simulink model "Motor_EncRead_AnalogRead"  (R2023a)
settings: Solver=ode3  StartTime=0.0  StopTime=inf  RelTol=1e-3  EnableMultiTasking=on
undefined symbols (not defined in the file or in its folder): ticksPerRot, wheelR
libraries: M5Core_Library x4, arduinolib x1
settings Model: ExtModeTrigDuration=2  Creator=auw_a  LastModifiedBy=auw_a
settings SolverCC: AlgebraicLoopSolver=TrustRegion
settings DataIOCC: LimitDataPoints=on  SaveFormat=Array
settings OptimizationCC: ExpressionDepthLimit=2147483647  LifeSpan=Inf  MaxStackSize=64
settings DebuggingCC: UnderspecifiedInitializationDetection=Classic  MergeDetectMultiDrivingBlocksExec=none  FcnCallInpInsideContextMsg=warning  UnconnectedInputMsg=warning  UnconnectedOutputMsg=warning  UnconnectedLineMsg=warning  AllowSymbolicDim=off  StateNameClashWarn=warning  SFUnexpectedBacktrackingDiag=warning  SFNoUnconditionalDefaultTransitionDiag=warning  SFExecutionAtInitializationDiag=none  ArithmeticOperatorsInVariantConditions=warning
settings HardwareCC: ProdBitPerPointer=32  ProdBitPerSizeT=32  ProdBitPerPtrDiffT=32  ProdLargestAtomicInteger=Long  ProdLargestAtomicFloat=Double  ProdWordSize=32  ProdHWDeviceType=ARM Compatible->ARM Cortex
settings ModelReferenceCC: EnableRefExpFcnMdlSchedulingChecks=on  PropagateSignalLabelsOutOfModel=off
settings SFSimCC: SimUseLocalCustomCode=off  CustomCodeUndefinedFunction=UseInterfaceOnly
settings RTWCC: Description=Embedded Coder  SystemTargetFile=ert.tlc  HardwareBoard=ESP32-WROOM(Arduino Compatible)  TemplateMakefile=ert_default_tmf  GenerateReport=on  RTWVerbose=off  RTWUseLocalCustomCode=off  Toolchain=ESP32  BuildConfiguration=Faster Runs  LaunchReport=on
settings CodeAppCC: ForceParamTrailComments=on  OperatorAnnotations=on  StateflowObjectComments=on  MATLABSourceComments=on
settings ERTTargetCC: MultiwordLength=2048  ERTCustomFileBanners=off  SupportContinuousTime=on  SupportNonInlinedSFcns=on  RemoveResetFunc=off  SupportVariableSizeSignals=on  ModelStepFunctionPrototypeControlCompliant=off  ExtModeTransport=3  ExtModeStaticAlloc=on  ExtModeAutomaticAllocSize=off  ExtModeStaticAllocSize=65536  ExtModeMexFile=ext_xcp  ExtModeIntrfLevel=Level2 - Open
settings ConfigComp: CovMetricSettings=dw  CovSaveCumulativeToWorkspaceVar=on  CovSaveSingleToWorkspaceVar=on  CovExternalEMLEnable=off  CovSFcnEnable=off

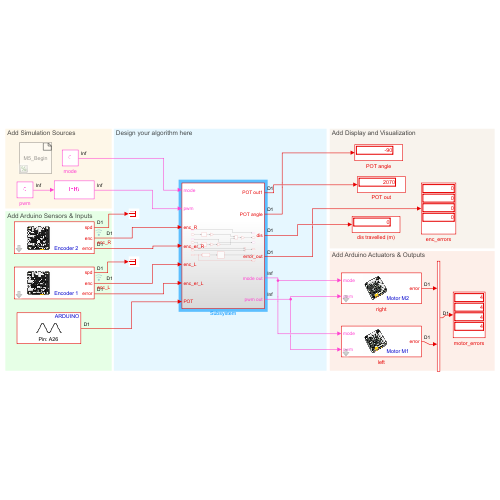
[thumbnail: Simulink's stored preview of the top-level diagram]
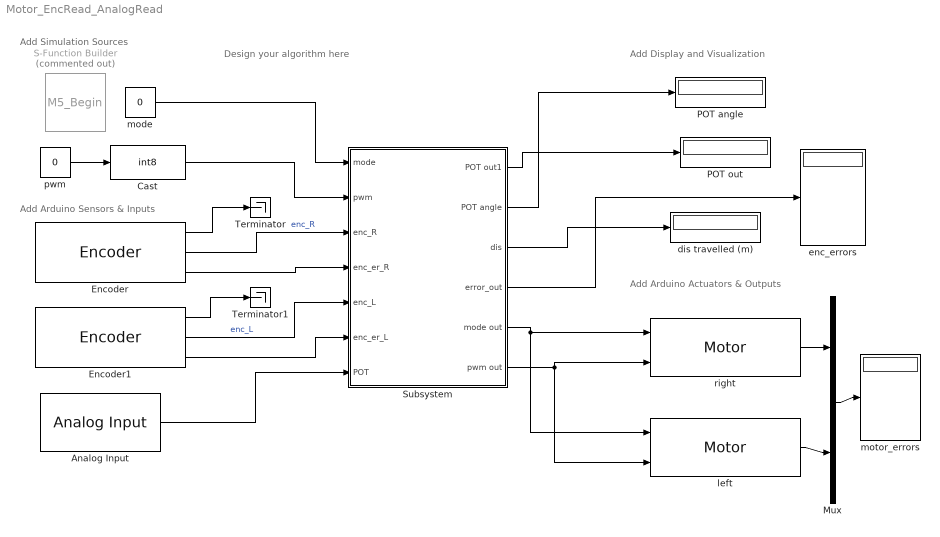
== system Motor_EncRead_AnalogRead ==
  note: Add Arduino Actuators & Outputs
  note: Add Arduino Sensors & Inputs
  note: Design your algorithm here
  note: Add Display and Visualization
  note: Add Simulation Sources
  Analog Input : arduinolib/Analog Input  pinNumber=26  ReadResultsOnly=off  ConversionTriggerSource=Software  ExternalTriggerType=uint32( 0 )  OutputDataType=uint16  EnableConversionCompleteNotify=off  EnableOuputStatus=off  SampleTime=0.01  blockPlatform=arduino
  Cast : DataTypeConversion  OutDataTypeStr=int8  SaturateOnIntegerOverflow=off  RndMeth=Floor
  Encoder : M5Core_Library/Encoder  M5_motor=2  s=0.01
      link override encoder I2C Read: RegisterAddress=uint8(hex2dec('40')) + m  SlaveDataType=int8
  Encoder1 : M5Core_Library/Encoder  M5_motor=1  s=0.01
  Mux : Mux  Inputs=2
  POT angle : Display
  POT out : Display
  S-Function Builder : S-Function  Commented=on  FunctionName=M5_Begin  SFunctionModules=M5_Begin_wrapper.cpp  SFunctionDeploymentMode=off  EnableBusSupport=off  mask(S-Function Builder){}
      mask help: Simulink:masks:SFunctionBuilder_MD
      mask init:
      | val = [[.9  0.75 0.75 1 1 .9 .9 1]',[1 1 0.75 0.75 .9 .9 1 .9]'];try , sys = get_param(gcb,'SfunBuilderFcnName');if isempty(sys), sys = get_param(gcb,'FunctionName'); end,catch, sys = get_param(gcb,'FunctionName'); end
      settings: CopyFcn=set_param(gcbh,'LinkStatus','none')  OpenFcn=sfunctionwizard(gcbh)
      mask Display:
      | plot(val(:,1),val(:,2))
      | disp(sys)
  Subsystem : Subsystem
  Terminator : Terminator
  Terminator1 : Terminator
  dis travelled (m) : Display
  enc_errors : Display
  left : M5Core_Library/Motor  M5_motor=M1
  mode : Constant  Value=0
  motor_errors : Display
  pwm : Constant  Value=0
  right : M5Core_Library/Motor  M5_motor=M2
  wires:
  pwm/1 -> Cast/1
  Encoder1/1 -> Terminator1/1
  Encoder/1 -> Terminator/1
  Encoder/2 -> Subsystem/3(enc_R)  "enc_R"
  Encoder1/2 -> Subsystem/5(enc_L)  "enc_L"
  mode/1 -> Subsystem/1(mode)
  Cast/1 -> Subsystem/2(pwm)
  Subsystem/5(mode out) -> left/1, right/1
  Encoder1/3 -> Subsystem/6(enc_er_L)
  Encoder/3 -> Subsystem/4(enc_er_R)
  Subsystem/3(dis) -> dis travelled (m)/1
  Analog Input/1 -> Subsystem/7(POT)
  Subsystem/2(POT angle) -> POT angle/1
  Subsystem/6(pwm out) -> right/2, left/2
  Subsystem/4(error_out) -> enc_errors/1
  right/1 -> Mux/1
  left/1 -> Mux/2
  Mux/1 -> motor_errors/1
  Subsystem/1(POT out1) -> POT out/1

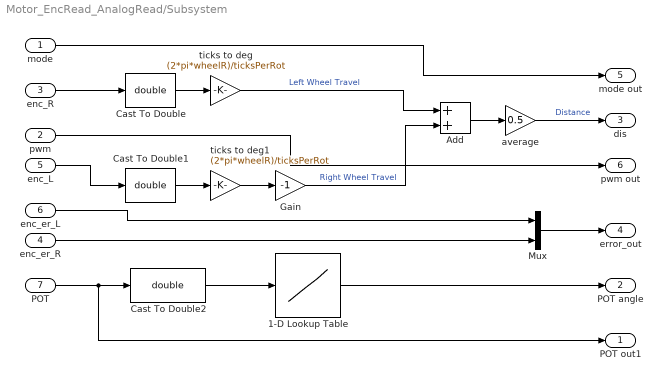
== system Motor_EncRead_AnalogRead/Subsystem ==
  mode : Inport
  pwm : Inport  Port=2
  enc_R : Inport  Port=3
  enc_er_R : Inport  Port=4
  enc_L : Inport  Port=5
  enc_er_L : Inport  Port=6
  POT : Inport  Port=7
  1-D Lookup Table : Lookup_n-D  NumberOfTableDimensions=1  BreakpointsForDimension1=linspace(2071,4095,180)  Table=linspace(90,-90,180)  ExtrapMethod=Clip  InternalRulePriority=Speed  RndMeth=Simplest
  Add : Sum
  Cast To Double : DataTypeConversion  OutDataTypeStr=double  SaturateOnIntegerOverflow=off  RndMeth=Floor
  Cast To Double1 : DataTypeConversion  OutDataTypeStr=double  SaturateOnIntegerOverflow=off  RndMeth=Floor
  Cast To Double2 : DataTypeConversion  OutDataTypeStr=double  SaturateOnIntegerOverflow=off  RndMeth=Floor
  Gain : Gain  Gain=-1
  Mux : Mux  Inputs=2
  average : Gain  Gain=0.5
  ticks to deg : Gain  Gain=(2*pi*wheelR)/ticksPerRot
  ticks to deg1 : Gain  Gain=(2*pi*wheelR)/ticksPerRot
  POT out1 : Outport
  POT angle : Outport  Port=2
  dis : Outport  Port=3
  error_out : Outport  Port=4
  mode out : Outport  Port=5
  pwm out : Outport  Port=6
  wires:
  Cast To Double/1 -> ticks to deg/1
  Gain/1 -> Add/2  "Right Wheel Travel"
  Cast To Double1/1 -> ticks to deg1/1
  Add/1 -> average/1
  ticks to deg/1 -> Add/1  "Left Wheel Travel"
  average/1 -> dis/1  "Distance"
  enc_L/1 -> Cast To Double1/1
  ticks to deg1/1 -> Gain/1
  enc_R/1 -> Cast To Double/1
  mode/1 -> mode out/1
  pwm/1 -> pwm out/1
  enc_er_L/1 -> Mux/1
  enc_er_R/1 -> Mux/2
  Mux/1 -> error_out/1
  POT/1 -> POT out1/1, Cast To Double2/1
  1-D Lookup Table/1 -> POT angle/1
  Cast To Double2/1 -> 1-D Lookup Table/1
